simulink subsystem "Controller"  (R2022b)
settings: Solver=VariableStepAuto  StartTime=0.0  StopTime=10.0  RelTol=1e-3
settings Model: Creator=Sahil Gaurkar  LastModifiedBy=Wikian

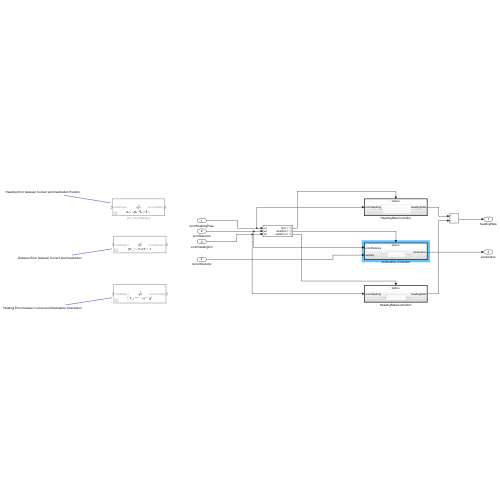
[thumbnail: Simulink's stored preview of the top-level diagram]
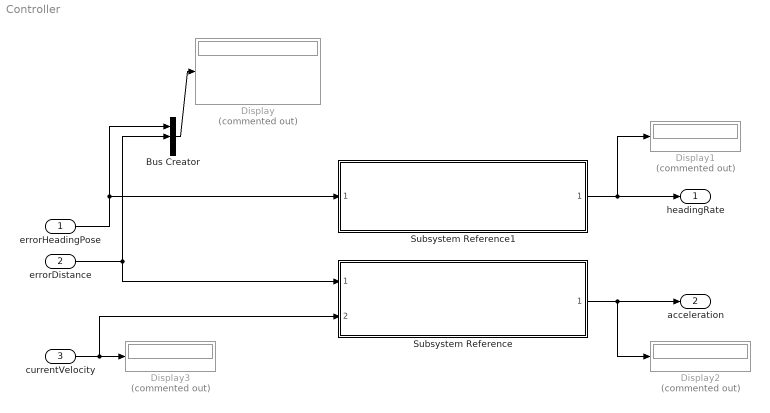
== system Controller ==
  errorHeadingPose : Inport
  errorDistance : Inport  Port=2
  currentVelocity : Inport  Port=3
  Bus Creator : BusCreator  Inputs=3
  Display{,1..3} (4 alike) : Display  Commented=on
  Subsystem Reference : Subsystem  ReferencedSubsystem=AcclerationController
  Subsystem Reference1 : Subsystem  ReferencedSubsystem=HeadingRateController
  headingRate : Outport
  acceleration : Outport  Port=2
  wires:
  errorDistance/1 -> Bus Creator/2, Subsystem Reference/1
  Subsystem Reference/1 -> acceleration/1, Display2/1
  Subsystem Reference1/1 -> headingRate/1, Display1/1
  currentVelocity/1 -> Display3/1, Subsystem Reference/2
  Bus Creator/1 -> Display/1
  errorHeadingPose/1 -> Subsystem Reference1/1, Bus Creator/1
